simulink model "silnik_wzor"  (R2017b)
settings: Solver=ode3  StartTime=0.0  StopTime=0.5  FixedStep=0.001  RelTol=1e-3  EnableMultiTasking=on
settings Model: Creator=Jacek  LastModifiedBy=mikos
settings DataIOCC: LimitDataPoints=on  SaveFormat=Array
settings OptimizationCC: LifeSpan=inf
settings DebuggingCC: SolverPrmCheckMsg=warning  SFUnexpectedBacktrackingDiag=warning  SFNoUnconditionalDefaultTransitionDiag=warning  SFExecutionAtInitializationDiag=none
settings HardwareCC: ProdBitPerPointer=32  ProdBitPerSizeT=32  ProdBitPerPtrDiffT=32  ProdLargestAtomicFloat=None  ProdIntDivRoundTo=Undefined  ProdEndianess=Unspecified  ProdWordSize=32  ProdHWDeviceType=32-bit Generic
settings ModelReferenceCC: PropagateSignalLabelsOutOfModel=off
settings CodeAppCC: StateflowObjectComments=on
settings GRTTargetCC: TargetLangStandard=C89/C90 (ANSI)
settings ConfigComp: CovMetricSettings=dw  CovSaveCumulativeToWorkspaceVar=on  CovSaveSingleToWorkspaceVar=on  CovExternalEMLEnable=off  CovSFcnEnable=off

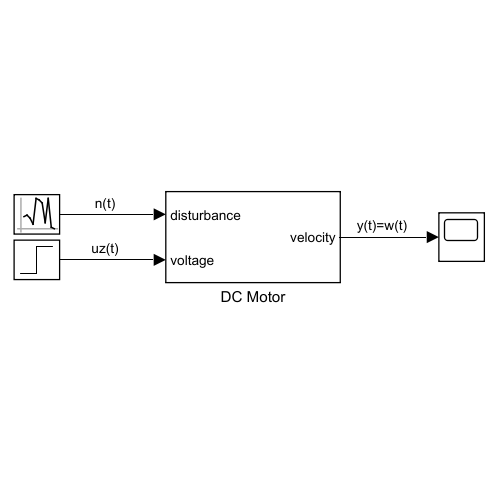
[thumbnail: Simulink's stored preview of the top-level diagram]
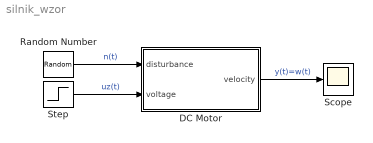
== system silnik_wzor ==
  DC Motor : Subsystem
  Random Number : RandomNumber  Variance=0
  Scope : Scope
  Step : Step  Time=0  After=300  SampleTime=0
  wires:
  Random Number/1 -> DC Motor/1(disturbance)  "n(t)"
  Step/1 -> DC Motor/2(voltage)  "uz(t)"
  DC Motor/1(velocity) -> Scope/1  "y(t)=w(t)"

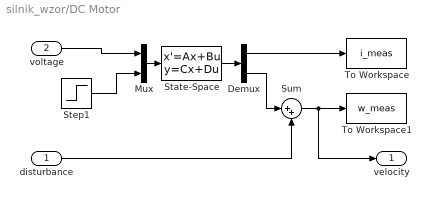
== system silnik_wzor/DC Motor ==
  disturbance : Inport
  voltage : Inport  Port=2
  Demux : Demux  Outputs=2
  Mux : Mux  Inputs=2
  State-Space : StateSpace  A=[-3/0.05, -2.23/0.05; 2.23/0.11, 0]  B=[1/0.05 0; 0 -1/0.11]  C=[1 0;0 1]  D=[0 0; 0 0]  InitialCondition=[0 ;40]
  Step1 : Step  Time=0.5  After=44.6  SampleTime=0
  Sum : Sum  Inputs=|++
  To Workspace : ToWorkspace  VariableName=i_meas  SampleTime=-1
  To Workspace1 : ToWorkspace  VariableName=w_meas  SampleTime=-1
  velocity : Outport  VectorParamsAs1DForOutWhenUnconnected=off
  wires:
  Mux/1 -> State-Space/1
  voltage/1 -> Mux/1
  Step1/1 -> Mux/2
  State-Space/1 -> Demux/1
  disturbance/1 -> Sum/2
  Demux/2 -> Sum/1
  Demux/1 -> To Workspace/1
  Sum/1 -> velocity/1, To Workspace1/1
